simulink model "defaultCtrlModel_2018a"  (R2018a)
settings: Solver=FixedStepAuto  StartTime=0.0  StopTime=200  FixedStep=Ts  RelTol=1e-3
values from neighbouring files (symbols this model uses):
  Kt = 0.882355004501468    (= 0.882355004501)    [initModels_GUI.m]
libraries: simulink x2
settings Model: Creator=Johannes  LastModifiedBy=HWRL user
settings SolverCC: ConcurrentTasks=on  PositivePriorityOrder=on
settings DataIOCC: ReturnWorkspaceOutputs=on
settings OptimizationCC: BlockReduction=off  OptimizeBlockIOStorage=off  ZeroExternalMemoryAtStartup=off
settings DebuggingCC: TasksWithSamePriorityMsg=none
settings HardwareCC: ProdBitPerLong=64  ProdLongLongMode=on  ProdHWDeviceType=Intel->x86-64 (Linux 64)
settings SFSimCC: SimUseLocalCustomCode=on
settings RTWCC: Description=Generic Real-Time Target  RTWUseLocalCustomCode=on  Toolchain=Simulink Real-Time Toolchain  BuildConfiguration=Faster Runs  TargetLang=C++
settings GRTTargetCC: TargetLangStandard=C++03 (ISO)  CodeInterfacePackaging=C++ class

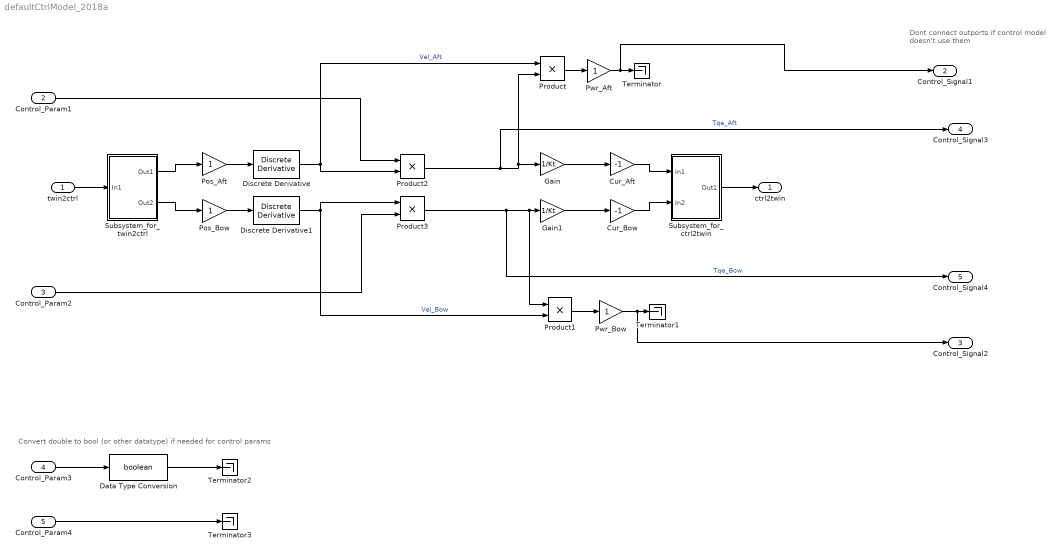
== system defaultCtrlModel_2018a ==
  note: Dont connect outports if control
      | model doesn't use them
  note: Convert double to bool (or other datatype) if needed for control params
  twin2ctrl : Inport
  Control_Param1 : Inport  Port=2
  Control_Param2 : Inport  Port=3
  Control_Param3 : Inport  Port=4  OutDataTypeStr=double
  Control_Param4 : Inport  Port=5  OutDataTypeStr=double
  Cur_Aft : Gain  Gain=-1
  Cur_Bow : Gain  Gain=-1
  Data Type Conversion : DataTypeConversion  OutDataTypeStr=boolean
  Discrete Derivative : simulink/Discrete/Discrete Derivative  gainval=1.0  ICPrevScaledInput=0.0  OutMin=[]  OutMax=[]  OutDataType=fixdt(1, 16)  OutScaling=2^-10  DoSatur=off
  Discrete Derivative1 : simulink/Discrete/Discrete Derivative  gainval=1.0  ICPrevScaledInput=0.0  OutMin=[]  OutMax=[]  OutDataType=fixdt(1, 16)  OutScaling=2^-10  DoSatur=off
  Gain : Gain  Gain=1/Kt
  Gain1 : Gain  Gain=1/Kt
  Pos_Aft : Gain
  Pos_Bow : Gain
  Product{,1..3} (4 alike) : Product
  Pwr_Aft : Gain
  Pwr_Bow : Gain
  Subsystem_for_ctrl2twin : Subsystem
  Subsystem_for_twin2ctrl : Subsystem
  Terminator{,1..3} (4 alike) : Terminator
  ctrl2twin : Outport
  Control_Signal1 : Outport  Port=2
  Control_Signal2 : Outport  Port=3
  Control_Signal3 : Outport  Port=4
  Control_Signal4 : Outport  Port=5
  wires:
  Pos_Aft/1 -> Discrete Derivative/1
  Discrete Derivative/1 -> Product/1, Product2/2  "Vel_Aft"
  Product3/1 -> Control_Signal4/1, Product1/1, Gain1/1  "Tqe_Bow"
  Discrete Derivative1/1 -> Product3/1, Product1/2  "Vel_Bow"
  Gain1/1 -> Cur_Bow/1
  Product1/1 -> Pwr_Bow/1
  Pwr_Bow/1 -> Control_Signal2/1, Terminator1/1
  Product/1 -> Pwr_Aft/1
  Gain/1 -> Cur_Aft/1
  Pos_Bow/1 -> Discrete Derivative1/1
  Product2/1 -> Control_Signal3/1, Product/2, Gain/1  "Tqe_Aft"
  Pwr_Aft/1 -> Control_Signal1/1, Terminator/1
  Control_Param2/1 -> Product3/2
  Control_Param1/1 -> Product2/1
  Control_Param3/1 -> Data Type Conversion/1
  Data Type Conversion/1 -> Terminator2/1
  Control_Param4/1 -> Terminator3/1
  Subsystem_for_ctrl2twin/1(Out1) -> ctrl2twin/1
  twin2ctrl/1 -> Subsystem_for_twin2ctrl/1(In1)
  Subsystem_for_twin2ctrl/1(Out1) -> Pos_Aft/1
  Subsystem_for_twin2ctrl/2(Out2) -> Pos_Bow/1
  Cur_Aft/1 -> Subsystem_for_ctrl2twin/1(In1)
  Cur_Bow/1 -> Subsystem_for_ctrl2twin/2(In2)

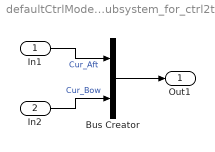
== system defaultCtrlModel_2018a/Subsystem_for_ctrl2twin ==
  In1 : Inport
  In2 : Inport  Port=2
  Bus Creator : BusCreator  Inputs=2
  Out1 : Outport
  wires:
  In1/1 -> Bus Creator/1  "Cur_Aft"
  In2/1 -> Bus Creator/2  "Cur_Bow"
  Bus Creator/1 -> Out1/1

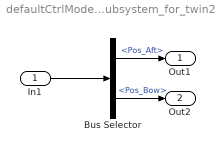
== system defaultCtrlModel_2018a/Subsystem_for_twin2ctrl ==
  In1 : Inport
  Bus Selector : BusSelector  OutputSignals=Pos_Aft,Pos_Bow
  Out1 : Outport
  Out2 : Outport  Port=2
  wires:
  In1/1 -> Bus Selector/1
  Bus Selector/1 -> Out1/1  "<Pos_Aft>"
  Bus Selector/2 -> Out2/1  "<Pos_Bow>"
